simulink model "QPSK_synch_demod"  (R2021a)
settings: Solver=VariableStepDiscrete  StartTime=0.0  StopTime=200000/fs  RelTol=1e-3  EnableMultiTasking=on
PreLoadFcn:
  | %%%%%%%%%%%%%%%%%%%%%%%%%%%%%%%%%%%%%%%%%%%%%%%%%%%%%%%%%%%%%%%%%%%%%%%%%%%
  | % check to see if Simulink library folder is missing from the MATLAB path %
  | %%%%%%%%%%%%%%%%%%%%%%%%%%%%%%%%%%%%%%%%%%%%%%%%%%%%%%%%%%%%%%%%%%%%%%%%%%%
  | if isempty(strfind(path, 'rtlsdr_book_library'))
  | 
  |     % create error window
  |     fig_error = figure(...
  |         'Name', 'Error: RTL-SDR Book Library',...
  |         'Toolbar','none',...
  |         'MenuBar','none',...
  |         'NumberTitle','off',...
  |         'Resize','off',...
  |         'WindowStyle','modal');
  |     fig_error.Position(3) = 600;
  |     fig_error.Position(4) = 150;
  |     fig_axes = axes(...
  |         'Parent',fig_error,...
  |         'Position',[0,0,1,1],...
  |         'visible','off');
  |     % error message
  |     t_title = text(.05,.8,...
  |         'MISSING DIRECTORIES',...
  |         'FontSize',11.5);
  |     t_body = text(.075,.6,...
  |         [{'Simulink cannot find the  \it{<root>}\rm / \it{rtlsdr\_book\_library}\rm  folder in the \it{MATLAB Path}\rm.'},...
  |         {'Please set the MATLAB path following the instructions given in Exercise 2.4.'}],...
  |         'FontSize',10.5);
  |     % buttons
  |     btn_path = uicontrol(...
  |         'Parent',fig_error,...
  |         'String','Set Path Now',...
  |         'FontSize',10,...
  |         'Callback', 'pathtool; close(fig_error);',...
  |         'Position', [fig_error.Position(3)/2-210, 30, 200, 30]);
  |     btn_abort = uicontrol(...
  |         'Parent',fig_error,...
  |         'String','No thanks',...
  |         'FontSize',10,...
  |         'Callback', 'close(fig_error); abort=1;',...
  |         'Position', [fig_error.Position(3)/2+10, 30, 200, 30]);
  | 
  |     % pause to allow user to interact with error box
  |     uiwait(fig_error);
  | 
  |     % abort simulation
  |     try
  |         if abort==1
  |             set_param(gcs, 'SimulationCommand', 'stop');
  |         end
  |     end
  | 
  |     % if user has set path, allow diagram to be updated
  |     if ~exist('abort','var')
  |         % create error window
  |         fig_update = figure(...
  |             'Name', 'Update Diagram',...
  |             'Toolbar','none',...
  |             'MenuBar','none',...
  |             'NumberTitle','off',...
  |             'Resize','off');
  |         fig_update.Position(3) = 400;
  |         fig_update.Position(4) = 120;
  |         fig_axes = axes(...
  |             'Parent',fig_update,...
  |             'Position',[0,0,1,1],...
  |             'visible','off');
  |         % instruction message
  |         t_body = text(.075,.7,...
  |             'Once you have set the path, update the block diagram',...
  |             'FontSize',10.5);
  |         % button
  |         btn_update = uicontrol(...
  |             'Parent',fig_update,...
  |             'String','Update Block Diagram',...
  |             'FontSize',10,...
  |             'Callback', 'set_param(gcs,''SimulationCommand'',''update''); close(gcf)',...
  |             'Position', [fig_update.Position(3)/2-100, 30, 200, 30]);
  |     end
  | 
  |     % clear error components
  |     clear('fig_error','fig_update','fig_axes','t_title','t_body','btn_path','btn_abort','btn_update','abort');
  | 
  | end
  | %%%%%%%%%%%%%%%%%%%%%%%%%%%%%%%%%%%%%%%%%%%%%%%%%%%%%%%%%%%%%%%%%%%%%%%%%%%
  | 
  | 
  | Rdata = 100e3;
  | Rsymbol = Rdata/2;
  | fs = 2.4e6;
  | MHz = fs/1e6;
  | interp = fs/Rsymbol;
  | fc = 600e3;
  | fe = 400;                     % frequency error at modulation
  | 
  | % ------- section for synch loop design --------
  | 
  | A = 1;       % assume input to loop has amplitude 1
  | 
  | T = 1/fs;        % sample period
  | Kp = A/2;       % phase detector S-curve is multiplier
  | Bn = 2000;    % noise bandwidth in Hz
  | Ko = 0.1;          % gain of NCO (here just a direct conversion)
  | 
  | d = 0.707;  % damping ratio
  | 
  | % calculate the loop filter coefficients
  | K1 = (4*d*Bn*T)/(Ko*Kp*(d+1/(4*d)));
  | K2 = (4*(Bn*T)^2)/(Ko*Kp*(d+1/4*d)^2);
undefined symbols (not defined in the file): startfcn_constellation
libraries: commfilt2 x4, commsynccomp2 x2, commrandsrc2 x1, rtlsdr_book_library x1, commdigbbndpm3 x1, dspsigops x1
CloseFcn:
  | closefcn_model;
Description:
  | Software, Simulation Examples and Design Exercises Licence Agreement
  | 
  | This license agreement refers to the simulation examples, design exercises and files,
  | and associated software MATLAB and Simulink resources that accompany the book:
  | 
  |      Title: Software Defined Radio using MATLAB & Simulink and the RTL-SDR
  |      Published by Strathclyde Academic Media, 2015
  |      Authored by Robert W. Stewart, Kenneth W. Barlee, Dale S.W. Atkinson,
  |      and Louise H. Crockett
  | 
  | and made available as a download from, www.desktopSDR.com or variously acquired
  | by other means such as via USB storage, cloud storage, disk or any other electronic
  | or optical or magnetic storage mechanism. These files and associated software may
  | be used subject to the terms of agreement of the conditions below:
  | 
  |     Copyright © 2015 Robert W. Stewart, Kenneth W. Barlee, Dale S.W. Atkinson,
  |     and Louise H. Crockett
  |     All rights reserved.
  | 
  | Redistribution and use in source and binary forms, with or without modification, are
  | permitted provided that the following conditions are met:
  | 
  |    1.  Redistributions of source code must retain the above copyright notice, this list of
  |         conditions and the following disclaimer.
  | 
  |    2.  Redistributions in binary form must reproduce the above copyright notice, this
  |         list of conditions and the following disclaimer in the documentation and/or other
  |         materials provided with the distribution.
  | 
  |    3.  Neither the name of the copyright holder nor the names of its contributors may
  |         be used to endorse or promote products derived from this software without
  |         specific prior written permission.
  | 
  |    4.  In all cases, the software is, and all modifications and derivatives of the
  |         software shall be, licensed to you solely for use in conjunction with The
  |         MathWorks, Inc. products and service offerings.
  | 
  | THIS SOFTWARE IS PROVIDED BY THE COPYRIGHT HOLDERS AND CONTRIBUTORS
  | "AS IS" AND ANY EXPRESS OR IMPLIED WARRANTIES, INCLUDING, BUT NOT LIMITED
  | TO, THE IMPLIED WARRANTIES OF MERCHANTABILITY AND FITNESS FOR A
  | PARTICULAR PURPOSE ARE DISCLAIMED. IN NO EVENT SHALL THE COPYRIGHT
  | HOLDER OR CONTRIBUTORS BE LIABLE FOR ANY DIRECT, INDIRECT, INCIDENTAL,
  | SPECIAL, EXEMPLARY, OR CONSEQUENTIAL DAMAGES (INCLUDING, BUT NOT
  | LIMITED TO, PROCUREMENT OF SUBSTITUTE GOODS OR SERVICES; LOSS OF USE,
  | DATA, OR PROFITS; OR BUSINESS INTERRUPTION) HOWEVER CAUSED AND ON ANY
  | THEORY OF LIABILITY, WHETHER IN CONTRACT, STRICT LIABILITY, OR TORT
  | (INCLUDING NEGLIGENCE OR OTHERWISE) ARISING IN ANY WAY OUT OF THE USE
  | OF THIS SOFTWARE, EVEN IF ADVISED OF THE POSSIBILITY OF SUCH DAMAGE.
  | 
  | 
  | Audio Tracks used in Simulations Examples and Design Exercises
  | 
  | The music and vocal files used within the Examples files and software within the book
  | were variously written, arranged, performed, recorded and produced by Garrey Rice,
  | Adam Struth, Jamie Struth, Iain Thistlethwaite and also Marshall Craigmyle who
  | collectively, and individually where appropriate, assert and retain all of their copyright,
  | performance and artistic rights. Permission to use and reproduce this music is
  | granted for all purposes associated with MATLAB and Simulink software and the
  | simulation examples and design exercises files that accompany this book. Requests to
  | use the music for any other purpose should be directed to: info@desktopSDR.com.
  | For information on music track names, full credits, and links to the musicians please
  | refer to www.desktopSDR.com/more/audio.
settings Model: Creator=desktopSDR Team  LastModifiedBy=liujiarun
settings SolverCC: AlgebraicLoopSolver=TrustRegion
settings DataIOCC: SaveFormat=Array  SaveOutput=off  SignalLogging=off  SaveTime=off  ReturnWorkspaceOutputs=off
settings OptimizationCC: LifeSpan=inf
settings DebuggingCC: UnderspecifiedInitializationDetection=Classic  MergeDetectMultiDrivingBlocksExec=none  SolverPrmCheckMsg=warning  SFUnexpectedBacktrackingDiag=warning  SFNoUnconditionalDefaultTransitionDiag=warning  SFExecutionAtInitializationDiag=none  SFMachineParentedDataDiag=warning  ArithmeticOperatorsInVariantConditions=warning
settings HardwareCC: ProdBitPerPointer=32  ProdBitPerSizeT=32  ProdBitPerPtrDiffT=32  ProdLargestAtomicFloat=None  ProdIntDivRoundTo=Undefined  ProdEndianess=Unspecified  ProdWordSize=32  ProdHWDeviceType=32-bit Generic
settings ModelReferenceCC: PropagateSignalLabelsOutOfModel=off
settings SFSimCC: SimUseLocalCustomCode=off  CustomCodeUndefinedFunction=UseInterfaceOnly
settings RTWCC: RTWUseLocalCustomCode=off
settings CodeAppCC: StateflowObjectComments=on
settings GRTTargetCC: TargetLangStandard=C89/C90 (ANSI)
settings ConfigComp: CovMetricSettings=dw  CovSaveCumulativeToWorkspaceVar=on  CovSaveSingleToWorkspaceVar=on  CovExternalEMLEnable=off  CovSFcnEnable=off

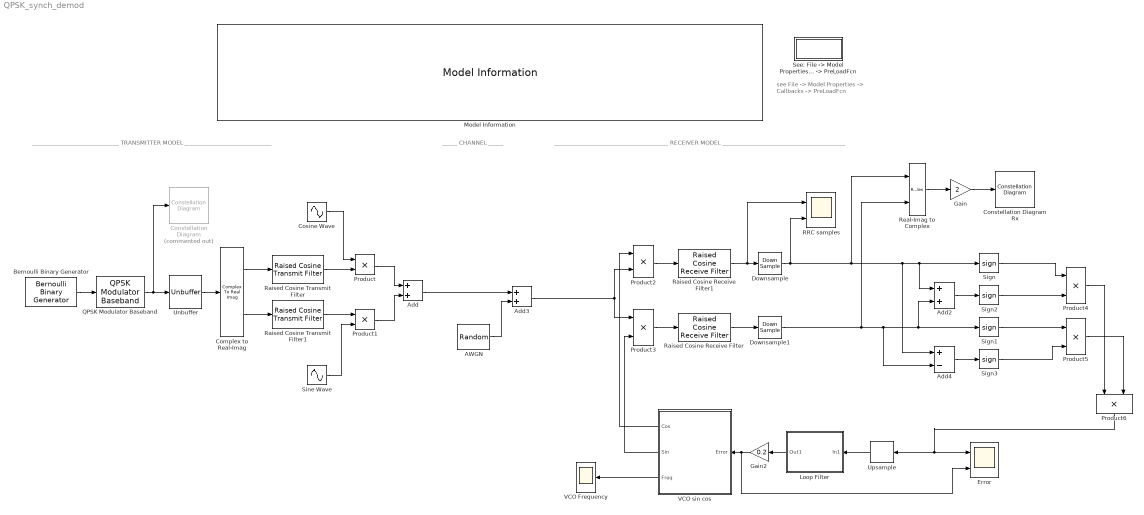
== system QPSK_synch_demod ==
  note: see File -> Model Properties
      | -> Callbacks -> PreLoadFcn
  note: _____________________________ TRANSMITTER MODEL _____________________________
  note: _____ CHANNEL _____
  note: ______________________________________ RECEIVER MODEL _________________________________________
  AWGN : RandomNumber  Variance=0.001  Seed=555  SampleTime=1/fs
  Add : Sum
  Add2 : Sum
  Add3 : Sum
  Add4 : Sum  Inputs=+-
  Bernoulli Binary Generator : commrandsrc2/Bernoulli Binary Generator  P=0.5  seed=61  Ts=1/Rdata  frameBased=on  sampPerFrame=2  orient=off  outDataType=double
      settings: SourceProductBaseCode=CM
  Complex to Real-Imag : ComplexToRealImag
  Constellation Diagram : ConstellationDiagram  Commented=on  StartFcn=startfcn_constellation;
  Constellation Diagram Rx : ConstellationDiagram  StartFcn=startfcn_constellation;
  Cosine Wave : Sin  Frequency=(fc+fe)*2*pi  Phase=pi/2  SampleTime=1/fs
  Downsample : DownSample  N=interp  RateOptions=Allow multirate processing
  Downsample1 : DownSample  N=interp  RateOptions=Allow multirate processing
  Error : Scope  NumInputPorts=2
      settings: StartFcn=startfcn_time_scope;
  Gain : Gain  Gain=2
  Gain2 : Gain  Gain=0.2
  Loop Filter : Subsystem
  Model Information : rtlsdr_book_library/Additional Tools/Model Information/Model Information
      settings: SourceProductName=RTL-SDR Book Library
  Product{,1..6} (7 alike) : Product
  QPSK Modulator Baseband : commdigbbndpm3/QPSK Modulator Baseband  InType=Bit  Enc=Gray  Ph=pi/4  outDtype=double  outWordLen=16  outUDDataType=sfix(16)  outFracLenMode=Best precision  outFracLen=15  outDataTypeStr=double  outLastDataTypeStr=double
  RRC samples : Scope  NumInputPorts=2
      settings: StartFcn=startfcn_time_scope;
  Raised Cosine Receive Filter : commfilt2/Raised Cosine Receive Filter  filtType=Square root  R=0.25  filtSpan=8  N=interp  downFactor=1  downOffset=0  filterGain=1  RateOptions=Allow multirate processing  framing=Allow multirate processing  checkCoeff=off  variableName=rcRxFilt  currentFiltSpan=8  D=(8)/2  inputOffset=0  sampMode=Mute  saveAsFlag=0  rateMode=Downsampling  checkGain=Normalized  launchFVT=on  roundingMode=Floor  overflowMode=off  coeffDataTypeStr=Inherit: Same word length as input  coeffMin=[]  coeffMax=[]  coeffLastDataTypeStr=Inherit: Same word length as input  accumDataTypeStr=Inherit: Same as product output  accumLastDataTypeStr=Inherit: Same as product output  outputDataTypeStr=Inherit: Same as accumulator  outputMin=[]  outputMax=[]  outputLastDataTypeStr=Inherit: Same as accumulator
  Raised Cosine Receive Filter1 : commfilt2/Raised Cosine Receive Filter  filtType=Square root  R=0.25  filtSpan=8  N=interp  downFactor=1  downOffset=0  filterGain=1  RateOptions=Allow multirate processing  framing=Allow multirate processing  checkCoeff=off  variableName=rcRxFilt1  currentFiltSpan=8  D=(8)/2  inputOffset=0  sampMode=Mute  saveAsFlag=0  rateMode=Downsampling  checkGain=Normalized  launchFVT=on  roundingMode=Floor  overflowMode=off  coeffDataTypeStr=Inherit: Same word length as input  coeffMin=[]  coeffMax=[]  coeffLastDataTypeStr=Inherit: Same word length as input  accumDataTypeStr=Inherit: Same as product output  accumLastDataTypeStr=Inherit: Same as product output  outputDataTypeStr=Inherit: Same as accumulator  outputMin=[]  outputMax=[]  outputLastDataTypeStr=Inherit: Same as accumulator
  Raised Cosine Transmit Filter : commfilt2/Raised Cosine Transmit Filter  filtType=Square root  R=0.25  filtSpan=8  N=interp  filterGain=1  RateOptions=Allow multirate processing  framing=Allow multirate processing  checkCoeff=off  variableName=rcTxFilt  checkGain=Normalized  sampMode=Mute  saveAsFlag=0  currentFiltSpan=8  D=(8)/2  launchFVT=on  roundingMode=Floor  overflowMode=off  coeffDataTypeStr=Inherit: Same word length as input  coeffMin=[]  coeffMax=[]  coeffLastDataTypeStr=Inherit: Same word length as input  outputDataTypeStr=Inherit: Same as accumulator  outputMin=[]  outputMax=[]  outputLastDataTypeStr=Inherit: Same as accumulator
  Raised Cosine Transmit Filter1 : commfilt2/Raised Cosine Transmit Filter  filtType=Square root  R=0.25  filtSpan=8  N=interp  filterGain=1  RateOptions=Allow multirate processing  framing=Allow multirate processing  checkCoeff=off  variableName=rcTxFilt1  checkGain=Normalized  sampMode=Mute  saveAsFlag=0  currentFiltSpan=8  D=(8)/2  launchFVT=on  roundingMode=Floor  overflowMode=off  coeffDataTypeStr=Inherit: Same word length as input  coeffMin=[]  coeffMax=[]  coeffLastDataTypeStr=Inherit: Same word length as input  outputDataTypeStr=Inherit: Same as accumulator  outputMin=[]  outputMax=[]  outputLastDataTypeStr=Inherit: Same as accumulator
  Real-Imag to Complex : RealImagToComplex
  "See: File -> Model Properties -> Callbacks -> PreLoadFcn " : Subsystem
      mask Display:
      | MHz = evalin('base', 'MHz');
      | fprintf(['fs = ',num2str(MHz),' MHz']);
  Sign{,1..3} (4 alike) : Signum  ZeroCross=off
  Sine Wave : Sin  Frequency=(fc+fe)*2*pi  SampleTime=1/fs
  Unbuffer : Unbuffer
  Upsample : dspsigops/Upsample  N=interp  phase=0  RateOptions=Allow multirate processing  ic=0  mode=Unused parameter value
  VCO Frequency : Scope
      settings: StartFcn=startfcn_time_scope;
  VCO sin cos : Subsystem  mask(Quadratude VCO){fq=fc, sensitivity=Ko*fs}
      mask prompts: fq "Quiescent Frequency (Hz)"; sensitivity "Sensitivity (Hz/V)"
      mask help: This VCO provides both cosine and sine outputs. The quiescent frequency and sensitivity of the VCO can be defined via the mask (and these apply to both sine and cosine outputs). The block also provides the instantaneous frequency as an output.
  wires:
  Bernoulli Binary Generator/1 -> QPSK Modulator Baseband/1
  QPSK Modulator Baseband/1 -> Unbuffer/1, Constellation Diagram/1
  Complex to Real-Imag/1 -> Raised Cosine Transmit Filter/1
  Complex to Real-Imag/2 -> Raised Cosine Transmit Filter1/1
  Raised Cosine Transmit Filter/1 -> Product/2
  Raised Cosine Transmit Filter1/1 -> Product1/1
  Sine Wave/1 -> Product1/2
  Unbuffer/1 -> Complex to Real-Imag/1
  Cosine Wave/1 -> Product/1
  VCO sin cos/1(Cos) -> Product2/1
  Product2/1 -> Raised Cosine Receive Filter1/1
  Product3/1 -> Raised Cosine Receive Filter/1
  Raised Cosine Receive Filter/1 -> Downsample1/1
  Raised Cosine Receive Filter1/1 -> RRC samples/1, Downsample/1
  Real-Imag to Complex/1 -> Gain/1
  Gain/1 -> Constellation Diagram Rx/1
  Product/1 -> Add/1
  Product1/1 -> Add/2
  VCO sin cos/3(Freq) -> VCO Frequency/1
  Upsample/1 -> Loop Filter/1(In1)
  Add/1 -> Add3/1
  Add3/1 -> Product2/2, Product3/1
  VCO sin cos/2(Sin) -> Product3/2
  Product4/1 -> Product6/1
  Product5/1 -> Product6/2
  Add2/1 -> Sign2/1
  Add4/1 -> Sign3/1
  Loop Filter/1(Out1) -> Gain2/1
  Gain2/1 -> Error/2, VCO sin cos/1(Error)
  Downsample/1 -> Add4/1, Sign/1, Add2/1, Real-Imag to Complex/1, RRC samples/2
  Downsample1/1 -> Add4/2, Add2/2, Sign1/1, Real-Imag to Complex/2
  Product6/1 -> Upsample/1, Error/1
  Sign2/1 -> Product4/2
  Sign1/1 -> Product5/1
  Sign3/1 -> Product5/2
  Sign/1 -> Product4/1
  AWGN/1 -> Add3/2

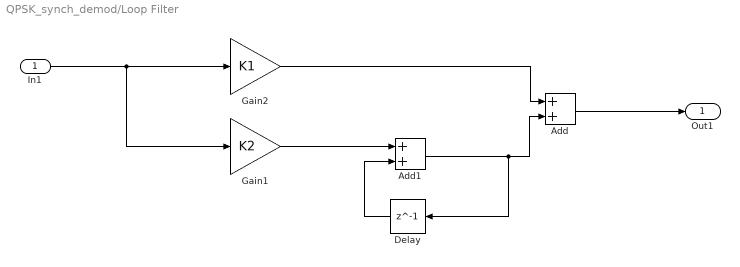
== system QPSK_synch_demod/Loop Filter ==
  In1 : Inport
  Add : Sum
  Add1 : Sum
  Delay : Delay  DelayLength=1
  Gain1 : Gain  Gain=K2
  Gain2 : Gain  Gain=K1
  Out1 : Outport
  wires:
  In1/1 -> Gain1/1, Gain2/1
  Add/1 -> Out1/1
  Gain2/1 -> Add/1
  Delay/1 -> Add1/2
  Gain1/1 -> Add1/1
  Add1/1 -> Delay/1, Add/2

== system QPSK_synch_demod/See: File -> Model Properties -> Callbacks -> PreLoadFcn  ==

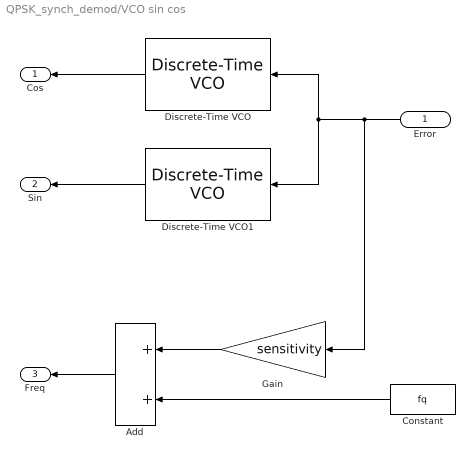
== system QPSK_synch_demod/VCO sin cos ==
  Error : Inport
  Add : Sum
  Constant : Constant  Value=fq  SampleTime=1/fs
  Discrete-Time VCO : commsynccomp2/Discrete-Time VCO  Ac=1  Fc=fq  Kc=sensitivity  Ph=pi/2  ts=1/fs
      settings: SourceProductBaseCode=CM
  Discrete-Time VCO1 : commsynccomp2/Discrete-Time VCO  Ac=1  Fc=fq  Kc=sensitivity  Ph=0  ts=1/fs
      settings: SourceProductBaseCode=CM
  Gain : Gain  Gain=sensitivity
  Cos : Outport
  Sin : Outport  Port=2
  Freq : Outport  Port=3
  wires:
  Discrete-Time VCO1/1 -> Sin/1
  Discrete-Time VCO/1 -> Cos/1
  Error/1 -> Gain/1, Discrete-Time VCO1/1, Discrete-Time VCO/1
  Gain/1 -> Add/1
  Constant/1 -> Add/2
  Add/1 -> Freq/1
